simulink model "Trabajo_final_PID"  (R2020a)
settings: Solver=VariableStepAuto  StartTime=0.0  StopTime=2.1  MaxStep=Ts3  RelTol=1e-3
values from neighbouring files (symbols this model uses):
  b_1 = 0    [param.m]
  b_2 = 0    [param.m]
  b_3 = 0    [param.m]
  b_4 = 0    [param.m]
  ba_1 = J_1 * omega_b * n    (= 0.00155)    [param.m]
  ba_2 = J_2 * omega_b * n    (= 0.00155)    [param.m]
  ba_3 = J_3 * omega_b * n    (= 0.000516666666667)    [param.m]
  ba_4 = J_4 * omega_b * n    (= 0.00031)    [param.m]
  J_1 = Jl    (= 3.1e-06)    [param.m]
  J_2 = Jl    (= 3.1e-06)    [param.m]
  J_3 = Jl/3    (= 1.03333333333e-06)    [param.m]
  J_4 = Jl/5    (= 6.2e-07)    [param.m]
  Ke_omega_1 = 3*(polo^2)    (= 1920000)    [param.m]
  Ke_omega_2 = 3*(polo^2)    (= 1920000)    [param.m]
  Ke_omega_3 = 3*(polo^2)    (= 1920000)    [param.m]
  Ke_omega_4 = 3*(polo^2)    (= 1920000)    [param.m]
  Ke_tita_1 = 3*polo    (= 2400)    [param.m]
  Ke_tita_2 = 3*polo    (= 2400)    [param.m]
  Ke_tita_3 = 3*polo    (= 2400)    [param.m]
  Ke_tita_4 = 3*polo    (= 2400)    [param.m]
  Ke_zeta_1 = polo^3    (= 512000000)    [param.m]
  Ke_zeta_2 = polo^3    (= 512000000)    [param.m]
  Ke_zeta_3 = polo^3    (= 512000000)    [param.m]
  Ke_zeta_4 = polo^3    (= 512000000)    [param.m]
  Ksa_1 = J_1 *n *omega_b^2    (= 0.31)    [param.m]
  Ksa_2 = J_2 *n *omega_b^2    (= 0.31)    [param.m]
  Ksa_3 = J_3 *n *omega_b^2    (= 0.103333333333)    [param.m]
  Ksa_4 = J_4 *n *omega_b^2    (= 0.062)    [param.m]
  Ksia_1 = J_1*omega_b^3    (= 24.8)    [param.m]
  Ksia_2 = J_2*omega_b^3    (= 24.8)    [param.m]
  Ksia_3 = J_3*omega_b^3    (= 8.26666666667)    [param.m]
  Ksia_4 = J_4*omega_b^3    (= 4.96)    [param.m]
  r1 = 71.2    [param.m]
  r2 = 99.5    [param.m]
  r3 = 171    [param.m]
  r4 = 298    [param.m]
  Ts1 = (omega_b*25/(2*pi))^(-1)    (= 0.00125663706144)    [param.m]
  Ts2 = (polo*25/(2*pi))^(-1)    (= 0.000314159265359)    [param.m]
undefined symbols (not defined in the file or in its folder): DiscIntNeverNeededParam
libraries: dspstat3 x8, robotmaniplib x7, simulink x2
settings Model: Creator=Rodrigo  LastModifiedBy=Rodrigo

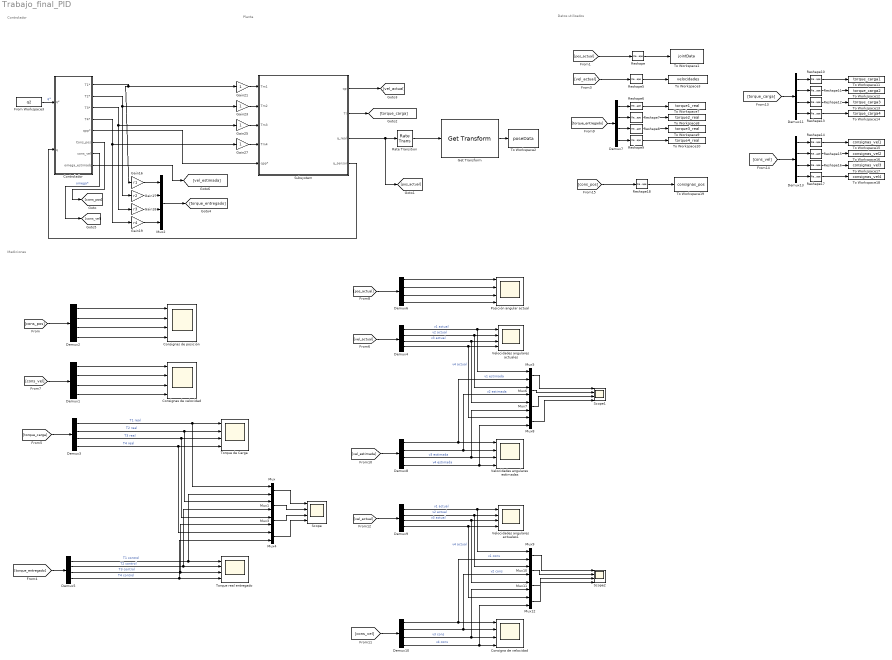
== system Trabajo_final_PID ==
  note: Planta
  note: Controlador
  note: Datos utilizados
  note: Mediciones
  "Consigna de velocidad " : Scope  NumInputPorts=4
  Consignas de posición : Scope  NumInputPorts=4
  Consignas de velocidad : Scope  NumInputPorts=4
  Controlador : Subsystem
  Demux{1..11,13} (12 alike) : Demux
  From Workspace3 : FromWorkspace  VariableName=q2  SampleTime=Ts2
  Gain16 : Gain  Gain=r1
  Gain17 : Gain  Gain=r2
  Gain18 : Gain  Gain=r3
  Gain19 : Gain  Gain=r4
  Gain{21,23,25,27} (4 alike) : Gain
  Get Transform : robotmaniplib/Get Transform  RigidBodyTree=robot  SourceBody=tool  TargetBody=base_link  SimulateUsing=Interpreted execution
  Mux{,1,3..12} (12 alike) : Mux  Inputs=2
  Mux2 : Mux
  Posición angular actual : Scope  NumInputPorts=4
  Rate Transition : RateTransition
  Reshape{,5..18} (15 alike) : Reshape
  Scope : Scope  NumInputPorts=4
  Scope1 : Scope  NumInputPorts=4
  Scope2 : Scope  NumInputPorts=4
  Subsystem : Subsystem
  To Workspace1 : ToWorkspace  VariableName=jointData  SampleTime=-1
      settings: Save2DSignal=2-D array (concatenate along first dimension)
  To Workspace10 : ToWorkspace  VariableName=torque4_real  SaveFormat=Timeseries  SampleTime=-1
  To Workspace11 : ToWorkspace  VariableName=torque_carga1  SaveFormat=Timeseries  SampleTime=-1
  To Workspace12 : ToWorkspace  VariableName=torque_carga2  SaveFormat=Timeseries  SampleTime=-1
  To Workspace13 : ToWorkspace  VariableName=torque_carga3  SaveFormat=Timeseries  SampleTime=-1
  To Workspace14 : ToWorkspace  VariableName=torque_carga4  SaveFormat=Timeseries  SampleTime=-1
  To Workspace15 : ToWorkspace  VariableName=consignas_vel1  SaveFormat=Timeseries  SampleTime=-1
  To Workspace16 : ToWorkspace  VariableName=consignas_vel2  SaveFormat=Timeseries  SampleTime=-1
  To Workspace17 : ToWorkspace  VariableName=consignas_vel3  SaveFormat=Timeseries  SampleTime=-1
  To Workspace18 : ToWorkspace  VariableName=consignas_vel4  SaveFormat=Timeseries  SampleTime=-1
  To Workspace19 : ToWorkspace  VariableName=consignas_pos  SampleTime=-1
      settings: Save2DSignal=2-D array (concatenate along first dimension)
  To Workspace2 : ToWorkspace  VariableName=poseData  SampleTime=-1
  To Workspace3 : ToWorkspace  VariableName=velocidades  SampleTime=-1
      settings: Save2DSignal=2-D array (concatenate along first dimension)
  To Workspace7 : ToWorkspace  VariableName=torque1_real  SaveFormat=Timeseries  SampleTime=-1
  To Workspace8 : ToWorkspace  VariableName=torque2_real  SaveFormat=Timeseries  SampleTime=-1
  To Workspace9 : ToWorkspace  VariableName=torque3_real  SaveFormat=Timeseries  SampleTime=-1
  Torque de Carga : Scope  NumInputPorts=4
  Torque real entregado : Scope  NumInputPorts=4
  Velocidades angulares actuales : Scope  NumInputPorts=4
  Velocidades angulares actuales1 : Scope  NumInputPorts=4
  Velocidades angulares estimadas : Scope  NumInputPorts=4
  wires:
  Rate Transition/1 -> Get Transform/1
  Get Transform/1 -> To Workspace2/1
  Demux2/1 -> Consignas de posición/1
  Demux2/2 -> Consignas de posición/2
  Demux2/3 -> Consignas de posición/3
  Demux2/4 -> Consignas de posición/4
  [cons_pos] -> Demux2/1
  Reshape/1 -> To Workspace1/1
  [pos_actual] -> Reshape/1
  Reshape5/1 -> To Workspace3/1
  [vel_actual] -> Reshape5/1
  Mux2/1 -> [torque_entregado]
  [torque_carga] -> Demux3/1
  Demux3/2 -> Torque de Carga/2, Mux1/1  "T2 real"
  Demux3/1 -> Torque de Carga/1, Mux/1  "T1 real"
  Demux3/3 -> Torque de Carga/3, Mux3/1  "T3 real"
  Demux3/4 -> Mux4/1, Torque de Carga/4  "T4 real"
  [vel_actual] -> Demux4/1
  Demux4/1 -> Mux5/1, Velocidades angulares actuales/1  "v1 actual"
  Demux4/2 -> Mux6/1, Velocidades angulares actuales/2  "v2 actual"
  Demux4/3 -> Mux7/1, Velocidades angulares actuales/3  "v3 actual"
  Demux4/4 -> Mux8/1, Velocidades angulares actuales/4  "v4 actual"
  [torque_entregado] -> Demux5/1
  Demux5/1 -> Torque real entregado/1, Mux/2  "T1 control"
  Demux5/2 -> Torque real entregado/2, Mux1/2  "T2 control"
  Demux5/3 -> Torque real entregado/3, Mux3/2  "T3 control"
  Demux5/4 -> Mux4/2, Torque real entregado/4  "T4 control"
  [cons_vel] -> Demux1/1
  Demux1/1 -> Consignas de velocidad/1
  Demux1/3 -> Consignas de velocidad/3
  Demux1/2 -> Consignas de velocidad/2
  Demux1/4 -> Consignas de velocidad/4
  Demux6/2 -> Posición angular actual/2
  [pos_actual] -> Demux6/1
  Demux6/4 -> Posición angular actual/4
  Demux6/1 -> Posición angular actual/1
  Demux6/3 -> Posición angular actual/3
  Reshape8/1 -> To Workspace9/1
  Demux7/2 -> Reshape7/1
  Demux7/4 -> Reshape9/1
  Reshape7/1 -> To Workspace8/1
  Reshape6/1 -> To Workspace7/1
  Reshape9/1 -> To Workspace10/1
  Demux7/1 -> Reshape6/1
  Demux7/3 -> Reshape8/1
  [torque_entregado] -> Demux7/1
  Gain19/1 -> Mux2/4
  Gain18/1 -> Mux2/3
  Gain17/1 -> Mux2/2
  Gain16/1 -> Mux2/1
  Gain25/1 -> Subsystem/3(Tm3)
  Gain27/1 -> Subsystem/4(Tm4)
  Gain23/1 -> Subsystem/2(Tm2)
  Gain21/1 -> Subsystem/1(Tm1)
  Subsystem/1(qp) -> [vel_actual]
  Subsystem/2(Tl) -> [torque_carga]
  Subsystem/3(q_real) -> [pos_actual], Rate Transition/1
  Controlador/4(T4*) -> Gain27/1, Gain19/1
  Controlador/3(T3*) -> Gain25/1, Gain18/1
  From Workspace3/1 -> Controlador/1(q*)  "q*"
  Controlador/2(T2*) -> Gain17/1, Gain23/1
  Controlador/5(qpp*) -> Subsystem/5(qpp*)
  Controlador/6(Cons_pos) -> [cons_pos]
  Controlador/7(cons_vel) -> [cons_vel]  "omega*"
  Controlador/1(T1*) -> Gain21/1, Gain16/1
  Mux/1 -> Scope/1
  Mux1/1 -> Scope/2
  Mux3/1 -> Scope/3
  Mux4/1 -> Scope/4
  Controlador/8(omega_estimado) -> [vel_estimada]
  Demux8/4 -> Mux8/2, Velocidades angulares estimadas/4  "v4 estimada"
  [vel_estimada] -> Demux8/1
  Demux8/2 -> Velocidades angulares estimadas/2, Mux6/2  "v2 estimada"
  Demux8/3 -> Mux7/2, Velocidades angulares estimadas/3  "v3 estimada"
  Demux8/1 -> Velocidades angulares estimadas/1, Mux5/2  "v1 estimada"
  Mux8/1 -> Scope1/4
  Mux7/1 -> Scope1/3
  Mux5/1 -> Scope1/1
  Mux6/1 -> Scope1/2
  [cons_vel] -> Demux10/1
  Demux10/1 -> "Consigna de velocidad "/1, Mux9/2  "v1 cons"
  Demux10/3 -> Mux11/2, "Consigna de velocidad "/3  "v3 cons"
  Demux10/4 -> Mux12/2, "Consigna de velocidad "/4  "v4 cons"
  Mux12/1 -> Scope2/4
  Demux10/2 -> "Consigna de velocidad "/2, Mux10/2  "v2 cons"
  Mux9/1 -> Scope2/1
  [vel_actual] -> Demux9/1
  Mux11/1 -> Scope2/3
  Demux9/3 -> Mux11/1, Velocidades angulares actuales1/3  "v3 actual"
  Demux9/2 -> Mux10/1, Velocidades angulares actuales1/2  "v2 actual"
  Demux9/1 -> Mux9/1, Velocidades angulares actuales1/1  "v1 actual"
  Mux10/1 -> Scope2/2
  Demux9/4 -> Mux12/1, Velocidades angulares actuales1/4  "v4 actual"
  Subsystem/4(q_sensor) -> Controlador/2(q)
  Reshape11/1 -> To Workspace12/1
  Reshape12/1 -> To Workspace13/1
  Demux11/2 -> Reshape11/1
  [torque_carga] -> Demux11/1
  Reshape10/1 -> To Workspace11/1
  Reshape13/1 -> To Workspace14/1
  Demux11/4 -> Reshape13/1
  Demux11/1 -> Reshape10/1
  Demux11/3 -> Reshape12/1
  Demux13/2 -> Reshape15/1
  Reshape14/1 -> To Workspace15/1
  Demux13/3 -> Reshape16/1
  [cons_vel] -> Demux13/1
  Reshape17/1 -> To Workspace18/1
  Reshape15/1 -> To Workspace16/1
  Demux13/1 -> Reshape14/1
  Demux13/4 -> Reshape17/1
  Reshape16/1 -> To Workspace17/1
  [cons_pos] -> Reshape18/1
  Reshape18/1 -> To Workspace19/1

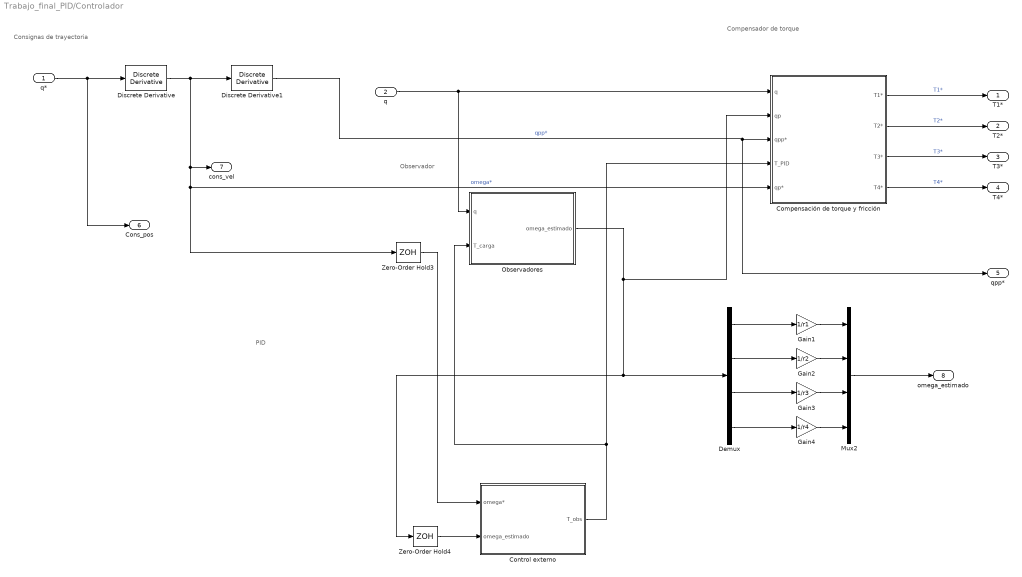
== system Trabajo_final_PID/Controlador ==
  note: Compensador de torque
  note: Observador
  note: PID
  note: Consignas de trayectoria
  q* : Inport
  q : Inport  Port=2
  Compensación de torque y fricción : Subsystem
  Control externo : Subsystem
  Demux : Demux
  Discrete Derivative : simulink/Discrete/Discrete Derivative  gainval=1.0  ICPrevScaledInput=0.0  OutMin=[]  OutMax=[]  OutDataType=fixdt(1, 16)  OutScaling=2^-10  DoSatur=off
  Discrete Derivative1 : simulink/Discrete/Discrete Derivative  gainval=1.0  ICPrevScaledInput=0.0  OutMin=[]  OutMax=[]  OutDataType=fixdt(1, 16)  OutScaling=2^-10  DoSatur=off
  Gain1 : Gain  Gain=1/r1
  Gain2 : Gain  Gain=1/r2
  Gain3 : Gain  Gain=1/r3
  Gain4 : Gain  Gain=1/r4
  Mux2 : Mux
  Observadores : Subsystem
  Zero-Order Hold3 : ZeroOrderHold  SampleTime=Ts1
  Zero-Order Hold4 : ZeroOrderHold  SampleTime=Ts1
  T1* : Outport
  T2* : Outport  Port=2
  T3* : Outport  Port=3
  T4* : Outport  Port=4
  qpp* : Outport  Port=5
  Cons_pos : Outport  Port=6
  cons_vel : Outport  Port=7
  omega_estimado : Outport  Port=8
  wires:
  Discrete Derivative/1 -> cons_vel/1, Zero-Order Hold3/1, Compensación de torque y fricción/5(qp*), Discrete Derivative1/1  "omega*"
  q/1 -> Compensación de torque y fricción/1(q), Observadores/1(q)
  Control externo/1(T_obs) -> Compensación de torque y fricción/4(T_PID), Observadores/2(T_carga)
  Discrete Derivative1/1 -> qpp*/1, Compensación de torque y fricción/3(qpp*)  "qpp*"
  Zero-Order Hold3/1 -> Control externo/1(omega*)
  Zero-Order Hold4/1 -> Control externo/2(omega_estimado)
  Compensación de torque y fricción/2(T2*) -> T2*/1  "T2*"
  Observadores/1(omega_estimado) -> Demux/1, Zero-Order Hold4/1, Compensación de torque y fricción/2(qp)
  Compensación de torque y fricción/4(T4*) -> T4*/1  "T4*"
  Compensación de torque y fricción/3(T3*) -> T3*/1  "T3*"
  Compensación de torque y fricción/1(T1*) -> T1*/1  "T1*"
  q*/1 -> Cons_pos/1, Discrete Derivative/1
  Gain2/1 -> Mux2/2
  Mux2/1 -> omega_estimado/1
  Gain1/1 -> Mux2/1
  Gain4/1 -> Mux2/4
  Gain3/1 -> Mux2/3
  Demux/1 -> Gain1/1
  Demux/2 -> Gain2/1
  Demux/3 -> Gain3/1
  Demux/4 -> Gain4/1

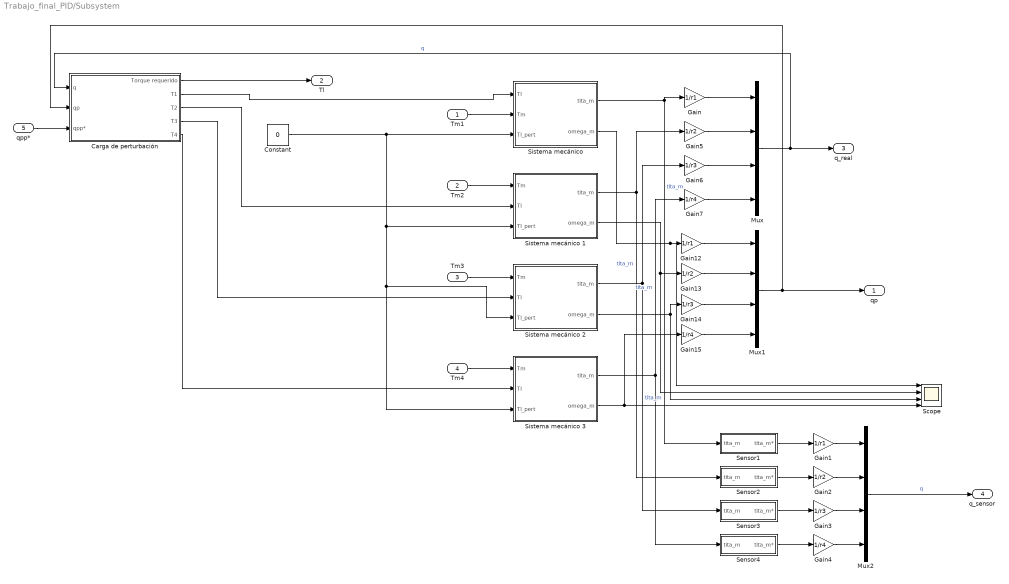
== system Trabajo_final_PID/Subsystem ==
  Tm1 : Inport
  Tm2 : Inport  Port=2
  Tm3 : Inport  Port=3
  Tm4 : Inport  Port=4
  qpp* : Inport  Port=5
  Carga de perturbación : Subsystem
  Constant : Constant  Value=0
  Gain : Gain  Gain=1/r1
  Gain1 : Gain  Gain=1/r1
  Gain12 : Gain  Gain=1/r1
  Gain13 : Gain  Gain=1/r2
  Gain14 : Gain  Gain=1/r3
  Gain15 : Gain  Gain=1/r4
  Gain2 : Gain  Gain=1/r2
  Gain3 : Gain  Gain=1/r3
  Gain4 : Gain  Gain=1/r4
  Gain5 : Gain  Gain=1/r2
  Gain6 : Gain  Gain=1/r3
  Gain7 : Gain  Gain=1/r4
  Mux : Mux
  Mux1 : Mux
  Mux2 : Mux
  Scope : Scope  NumInputPorts=4
  Sensor1 : Subsystem
  Sensor2 : Subsystem
  Sensor3 : Subsystem
  Sensor4 : Subsystem
  "Sistema mecánico " : Subsystem
  Sistema mecánico 1 : Subsystem
  Sistema mecánico 2 : Subsystem
  Sistema mecánico 3 : Subsystem
  qp : Outport
  Tl : Outport  Port=2
  q_real : Outport  Port=3
  q_sensor : Outport  Port=4
  wires:
  Gain13/1 -> Mux1/2
  Gain5/1 -> Mux/2
  Sistema mecánico 3/2(omega_m) -> Gain15/1, Scope/4
  Gain15/1 -> Mux1/4
  Sistema mecánico 3/1(tita_m) -> Sensor4/1(tita_m), Gain7/1  "tita_m"
  Mux/1 -> q_real/1, Carga de perturbación/1(q)  "q"
  Tm1/1 -> "Sistema mecánico "/2(Tm)
  Sistema mecánico 1/2(omega_m) -> Scope/2, Gain13/1
  Tm4/1 -> Sistema mecánico 3/1(Tm)
  "Sistema mecánico "/2(omega_m) -> Scope/1, Gain12/1
  Sistema mecánico 1/1(tita_m) -> Sensor2/1(tita_m), Gain5/1  "tita_m"
  Sistema mecánico 2/2(omega_m) -> Gain14/1, Scope/3
  Gain12/1 -> Mux1/1
  Gain14/1 -> Mux1/3
  Gain7/1 -> Mux/4
  Gain/1 -> Mux/1
  Gain6/1 -> Mux/3
  Sistema mecánico 2/1(tita_m) -> Sensor3/1(tita_m), Gain6/1  "tita_m"
  "Sistema mecánico "/1(tita_m) -> Gain/1, Sensor1/1(tita_m)  "tita_m"
  Tm3/1 -> Sistema mecánico 2/1(Tm)
  Tm2/1 -> Sistema mecánico 1/1(Tm)
  Carga de perturbación/2(T1) -> "Sistema mecánico "/1(Tl)
  Carga de perturbación/3(T2) -> Sistema mecánico 1/2(Tl)
  Carga de perturbación/4(T3) -> Sistema mecánico 2/2(Tl)
  Carga de perturbación/5(T4) -> Sistema mecánico 3/2(Tl)
  Carga de perturbación/1(Torque requerido) -> Tl/1
  Mux1/1 -> Carga de perturbación/2(qp), qp/1
  qpp*/1 -> Carga de perturbación/3(qpp*)
  Gain1/1 -> Mux2/1
  Sensor1/1(tita_m*) -> Gain1/1
  Gain2/1 -> Mux2/2
  Gain3/1 -> Mux2/3
  Gain4/1 -> Mux2/4
  Sensor4/1(tita_m*) -> Gain4/1
  Sensor3/1(tita_m*) -> Gain3/1
  Sensor2/1(tita_m*) -> Gain2/1
  Mux2/1 -> q_sensor/1  "q"
  Constant/1 -> Sistema mecánico 3/3(Tl_pert), Sistema mecánico 2/3(Tl_pert), Sistema mecánico 1/3(Tl_pert), "Sistema mecánico "/3(Tl_pert)

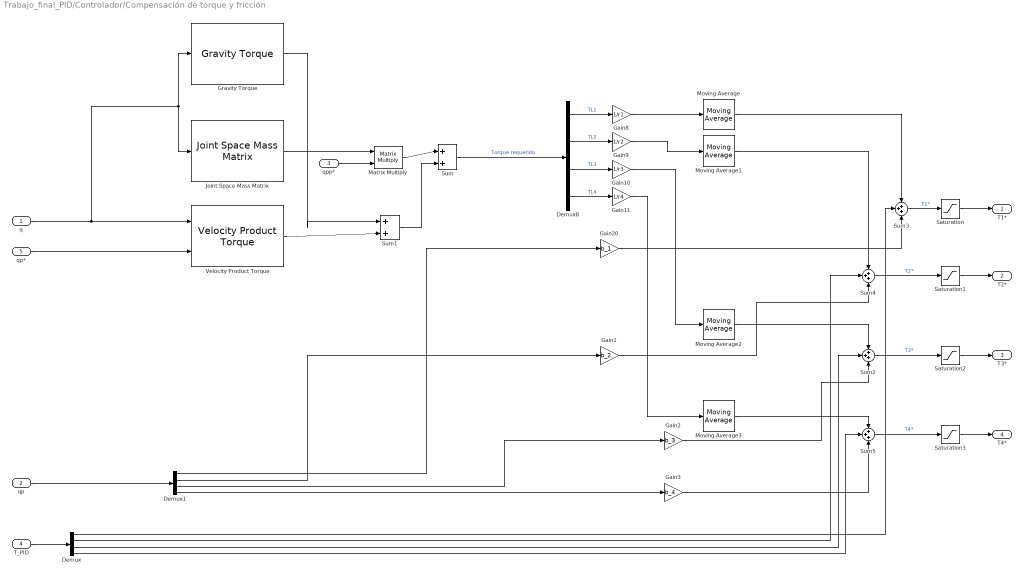
== system Trabajo_final_PID/Controlador/Compensación de torque y fricción ==
  q : Inport
  qp : Inport  Port=2
  qpp* : Inport  Port=3
  T_PID : Inport  Port=4
  qp* : Inport  Port=5
  Demux : Demux
  Demux1 : Demux
  Demux8 : Demux
  Gain1 : Gain  Gain=b_2
  Gain10 : Gain  Gain=1/r3
  Gain11 : Gain  Gain=1/r4
  Gain2 : Gain  Gain=b_3
  Gain20 : Gain  Gain=b_1
  Gain3 : Gain  Gain=b_4
  Gain8 : Gain  Gain=1/r1
  Gain9 : Gain  Gain=1/r2
  Gravity Torque : robotmaniplib/Gravity Torque  RigidBodyTree=robot  SimulateUsing=Interpreted execution
  Joint Space Mass Matrix : robotmaniplib/Joint Space Mass Matrix  RigidBodyTree=robot  SimulateUsing=Interpreted execution
  Matrix Multiply : Product  Multiplication=Matrix(*)
  Moving Average{,1..3} (4 alike) : dspstat3/Moving Average  Method=Sliding window  ForgettingFactorPort=off  SpecifyWindowLength=on  WindowLength=5  ForgettingFactor=0.9  SimulateUsing=Code generation
  Saturation : Saturate  UpperLimit=10/r1  LowerLimit=-10/r1
  Saturation1 : Saturate  UpperLimit=8.2/r2  LowerLimit=-8.2/r2
  Saturation2 : Saturate  UpperLimit=3/r3  LowerLimit=-3/r3
  Saturation3 : Saturate  UpperLimit=0.8/r4  LowerLimit=-0.8/r4
  Sum : Sum  Inputs=|++
  Sum1 : Sum  Inputs=|++
  Sum{2..5} (4 alike) : Sum  Inputs=+++
  Velocity Product Torque : robotmaniplib/Velocity Product Torque  RigidBodyTree=robot  SimulateUsing=Interpreted execution
      settings: SourceProductBaseCode=RO
  T1* : Outport
  T2* : Outport  Port=2
  T3* : Outport  Port=3
  T4* : Outport  Port=4
  wires:
  q/1 -> Velocity Product Torque/1, Gravity Torque/1, Joint Space Mass Matrix/1
  Demux8/1 -> Gain8/1  "TL1"
  Matrix Multiply/1 -> Sum/1
  Sum/1 -> Demux8/1  "Torque requerido"
  Gravity Torque/1 -> Sum1/1
  Velocity Product Torque/1 -> Sum1/2
  Joint Space Mass Matrix/1 -> Matrix Multiply/1
  Sum1/1 -> Sum/2
  Demux8/4 -> Gain11/1  "TL4"
  Demux8/3 -> Gain10/1  "TL3"
  Demux8/2 -> Gain9/1  "TL2"
  qpp*/1 -> Matrix Multiply/2
  qp/1 -> Demux1/1
  Sum2/1 -> Saturation2/1  "T3*"
  Saturation2/1 -> T3*/1
  Gain10/1 -> Moving Average2/1
  Gain9/1 -> Moving Average1/1
  Saturation1/1 -> T2*/1
  Sum3/1 -> Saturation/1  "T1*"
  Sum4/1 -> Saturation1/1  "T2*"
  Saturation/1 -> T1*/1
  Demux/1 -> Sum3/2
  Sum5/1 -> Saturation3/1  "T4*"
  Gain8/1 -> Moving Average/1
  Gain11/1 -> Moving Average3/1
  Saturation3/1 -> T4*/1
  Gain20/1 -> Sum3/3
  Gain1/1 -> Sum4/3
  Gain2/1 -> Sum2/3
  Gain3/1 -> Sum5/3
  Demux1/1 -> Gain20/1
  Demux1/2 -> Gain1/1
  Demux1/3 -> Gain2/1
  Demux1/4 -> Gain3/1
  Demux/2 -> Sum4/2
  Demux/3 -> Sum2/2
  Demux/4 -> Sum5/2
  T_PID/1 -> Demux/1
  Moving Average/1 -> Sum3/1
  Moving Average1/1 -> Sum4/1
  Moving Average2/1 -> Sum2/1
  Moving Average3/1 -> Sum5/1
  qp*/1 -> Velocity Product Torque/2

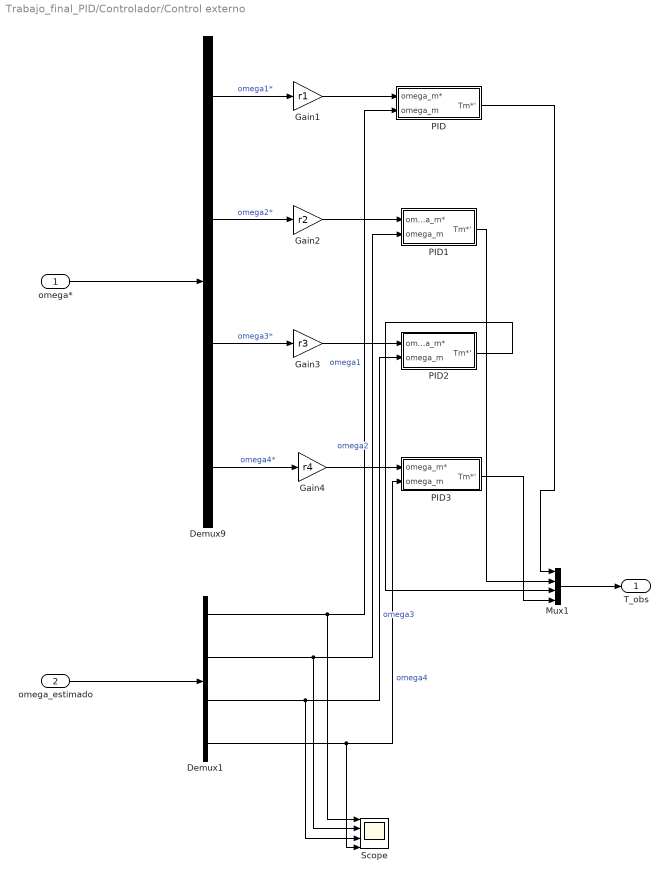
== system Trabajo_final_PID/Controlador/Control externo ==
  omega* : Inport
  omega_estimado : Inport  Port=2
  Demux1 : Demux
  Demux9 : Demux
  Gain1 : Gain  Gain=r1
  Gain2 : Gain  Gain=r2
  Gain3 : Gain  Gain=r3
  Gain4 : Gain  Gain=r4
  Mux1 : Mux
  PID : Subsystem
  PID1 : Subsystem
  PID2 : Subsystem
  PID3 : Subsystem
  Scope : Scope  NumInputPorts=4
  T_obs : Outport
  wires:
  Demux9/3 -> Gain3/1  "omega3*"
  Gain2/1 -> PID1/1(omega_m*)
  Gain3/1 -> PID2/1(omega_m*)
  Demux9/1 -> Gain1/1  "omega1*"
  Demux9/2 -> Gain2/1  "omega2*"
  Gain4/1 -> PID3/1(omega_m*)
  Demux9/4 -> Gain4/1  "omega4*"
  Gain1/1 -> PID/1(omega_m*)
  Demux1/2 -> Scope/2, PID1/2(omega_m)  "omega2"
  Demux1/1 -> Scope/1, PID/2(omega_m)  "omega1"
  Demux1/3 -> Scope/3, PID2/2(omega_m)  "omega3"
  Demux1/4 -> Scope/4, PID3/2(omega_m)  "omega4"
  PID/1(Tm*') -> Mux1/1
  PID1/1(Tm*') -> Mux1/2
  PID2/1(Tm*') -> Mux1/3
  PID3/1(Tm*') -> Mux1/4
  Mux1/1 -> T_obs/1
  omega*/1 -> Demux9/1
  omega_estimado/1 -> Demux1/1

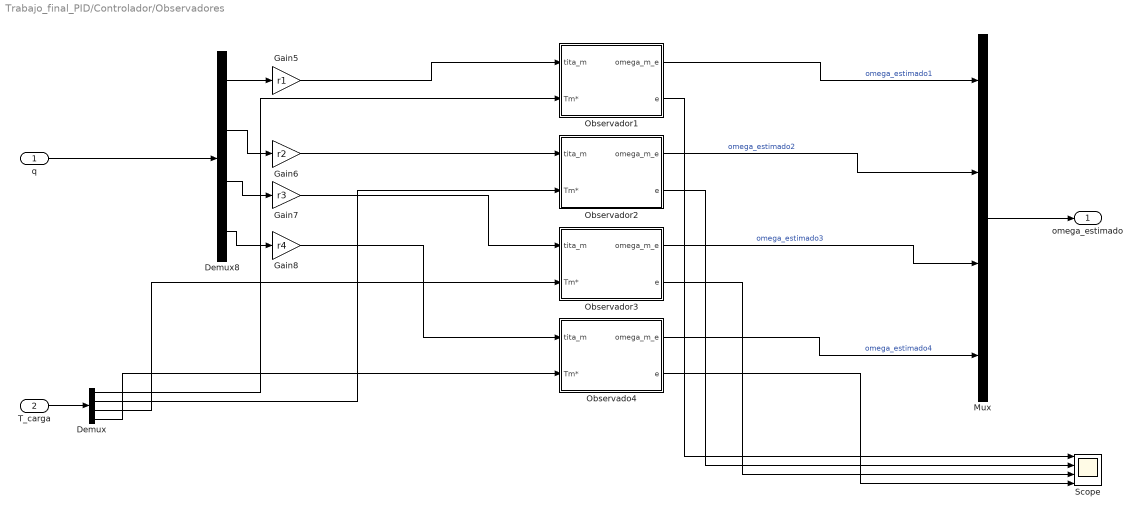
== system Trabajo_final_PID/Controlador/Observadores ==
  q : Inport
  T_carga : Inport  Port=2
  Demux : Demux
  Demux8 : Demux
  Gain5 : Gain  Gain=r1
  Gain6 : Gain  Gain=r2
  Gain7 : Gain  Gain=r3
  Gain8 : Gain  Gain=r4
  Mux : Mux
  Observado4 : Subsystem
  Observador1 : Subsystem
  Observador2 : Subsystem
  Observador3 : Subsystem
  Scope : Scope  NumInputPorts=4
  omega_estimado : Outport
  wires:
  Gain6/1 -> Observador2/1(tita_m)
  Demux8/3 -> Gain7/1
  Gain5/1 -> Observador1/1(tita_m)
  Demux8/1 -> Gain5/1
  Observador2/1(omega_m_e) -> Mux/2  "omega_estimado2"
  Demux8/2 -> Gain6/1
  Demux8/4 -> Gain8/1
  Gain7/1 -> Observador3/1(tita_m)
  Gain8/1 -> Observado4/1(tita_m)
  Observador1/1(omega_m_e) -> Mux/1  "omega_estimado1"
  Observado4/1(omega_m_e) -> Mux/4  "omega_estimado4"
  Observador3/1(omega_m_e) -> Mux/3  "omega_estimado3"
  q/1 -> Demux8/1
  Mux/1 -> omega_estimado/1
  T_carga/1 -> Demux/1
  Demux/1 -> Observador1/2(Tm*)
  Demux/2 -> Observador2/2(Tm*)
  Demux/3 -> Observador3/2(Tm*)
  Demux/4 -> Observado4/2(Tm*)
  Observador1/2(e) -> Scope/1
  Observador2/2(e) -> Scope/2
  Observador3/2(e) -> Scope/3
  Observado4/2(e) -> Scope/4

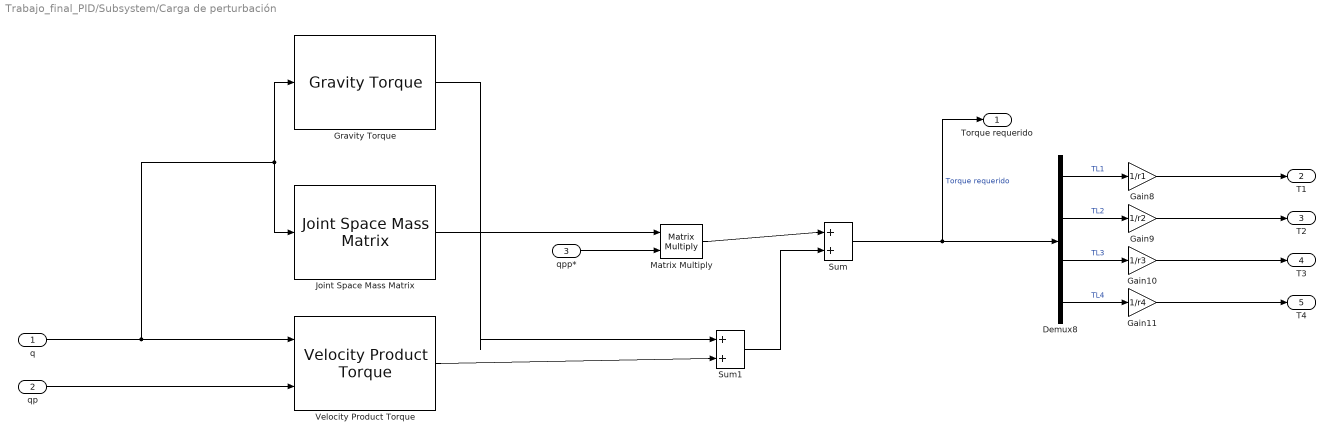
== system Trabajo_final_PID/Subsystem/Carga de perturbación ==
  q : Inport
  qp : Inport  Port=2
  qpp* : Inport  Port=3
  Demux8 : Demux
  Gain10 : Gain  Gain=1/r3
  Gain11 : Gain  Gain=1/r4
  Gain8 : Gain  Gain=1/r1
  Gain9 : Gain  Gain=1/r2
  Gravity Torque : robotmaniplib/Gravity Torque  RigidBodyTree=robot  SimulateUsing=Interpreted execution
  Joint Space Mass Matrix : robotmaniplib/Joint Space Mass Matrix  RigidBodyTree=robot  SimulateUsing=Interpreted execution
  Matrix Multiply : Product  Multiplication=Matrix(*)
  Sum : Sum  Inputs=|++
  Sum1 : Sum  Inputs=|++
  Velocity Product Torque : robotmaniplib/Velocity Product Torque  RigidBodyTree=robot  SimulateUsing=Interpreted execution
      settings: SourceProductBaseCode=RO
  Torque requerido : Outport
  T1 : Outport  Port=2
  T2 : Outport  Port=3
  T3 : Outport  Port=4
  T4 : Outport  Port=5
  wires:
  q/1 -> Velocity Product Torque/1, Gravity Torque/1, Joint Space Mass Matrix/1
  Demux8/1 -> Gain8/1  "TL1"
  Matrix Multiply/1 -> Sum/1
  Sum/1 -> Demux8/1, Torque requerido/1  "Torque requerido"
  Gravity Torque/1 -> Sum1/1
  Velocity Product Torque/1 -> Sum1/2
  Joint Space Mass Matrix/1 -> Matrix Multiply/1
  Sum1/1 -> Sum/2
  Demux8/4 -> Gain11/1  "TL4"
  Demux8/3 -> Gain10/1  "TL3"
  Gain11/1 -> T4/1
  Demux8/2 -> Gain9/1  "TL2"
  qpp*/1 -> Matrix Multiply/2
  qp/1 -> Velocity Product Torque/2
  Gain9/1 -> T2/1
  Gain8/1 -> T1/1
  Gain10/1 -> T3/1

== system Trabajo_final_PID/Subsystem/Sensor1 ==
  tita_m : Inport
  Moving Average : dspstat3/Moving Average  Method=Sliding window  ForgettingFactorPort=off  SpecifyWindowLength=on  WindowLength=8  ForgettingFactor=0.9  SimulateUsing=Code generation
  Quantizer : Quantizer  QuantizationInterval=int_encoder
  Random Number : RandomNumber  Variance=(1/360)^2  SampleTime=Ts2  VectorParams1D=off
  Sum : Sum  Inputs=|++
  Zero-Order Hold1 : ZeroOrderHold  SampleTime=Ts2
  tita_m* : Outport
  wires:
  tita_m/1 -> Quantizer/1
  Random Number/1 -> Sum/2
  Zero-Order Hold1/1 -> Moving Average/1  "tita_m*"
  Moving Average/1 -> tita_m*/1
  Sum/1 -> Zero-Order Hold1/1
  Quantizer/1 -> Sum/1

== system Trabajo_final_PID/Subsystem/Sensor2 ==
  tita_m : Inport
  Moving Average : dspstat3/Moving Average  Method=Sliding window  ForgettingFactorPort=off  SpecifyWindowLength=on  WindowLength=8  ForgettingFactor=0.9  SimulateUsing=Code generation
  Quantizer : Quantizer  QuantizationInterval=int_encoder
  Random Number : RandomNumber  Variance=(1/360)^2  SampleTime=Ts2  VectorParams1D=off
  Sum : Sum  Inputs=|++
  Zero-Order Hold1 : ZeroOrderHold  SampleTime=Ts2
  tita_m* : Outport
  wires:
  tita_m/1 -> Quantizer/1
  Random Number/1 -> Sum/2
  Sum/1 -> Zero-Order Hold1/1
  Zero-Order Hold1/1 -> Moving Average/1  "tita_m*"
  Moving Average/1 -> tita_m*/1
  Quantizer/1 -> Sum/1

== system Trabajo_final_PID/Subsystem/Sensor3 ==
  tita_m : Inport
  Moving Average : dspstat3/Moving Average  Method=Sliding window  ForgettingFactorPort=off  SpecifyWindowLength=on  WindowLength=8  ForgettingFactor=0.9  SimulateUsing=Code generation
  Quantizer : Quantizer  QuantizationInterval=int_encoder
  Random Number : RandomNumber  Variance=(1/360)^2  SampleTime=Ts2  VectorParams1D=off
  Sum : Sum  Inputs=|++
  Zero-Order Hold1 : ZeroOrderHold  SampleTime=Ts2
  tita_m* : Outport
  wires:
  tita_m/1 -> Quantizer/1
  Random Number/1 -> Sum/2
  Sum/1 -> Zero-Order Hold1/1
  Zero-Order Hold1/1 -> Moving Average/1  "tita_m*"
  Moving Average/1 -> tita_m*/1
  Quantizer/1 -> Sum/1

== system Trabajo_final_PID/Subsystem/Sensor4 ==
  tita_m : Inport
  Moving Average : dspstat3/Moving Average  Method=Sliding window  ForgettingFactorPort=off  SpecifyWindowLength=on  WindowLength=8  ForgettingFactor=0.9  SimulateUsing=Code generation
  Quantizer : Quantizer  QuantizationInterval=int_encoder
  Random Number : RandomNumber  Variance=(1/360)^2  SampleTime=Ts2  VectorParams1D=off
  Sum : Sum  Inputs=|++
  Zero-Order Hold1 : ZeroOrderHold  SampleTime=Ts2
  tita_m* : Outport
  wires:
  tita_m/1 -> Quantizer/1
  Random Number/1 -> Sum/2
  Sum/1 -> Zero-Order Hold1/1
  Zero-Order Hold1/1 -> Moving Average/1  "tita_m*"
  Moving Average/1 -> tita_m*/1
  Quantizer/1 -> Sum/1

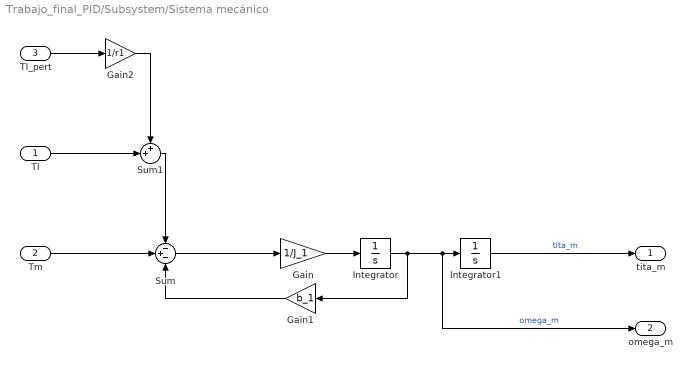
== system Trabajo_final_PID/Subsystem/Sistema mecánico  ==
  Tl : Inport
  Tm : Inport  Port=2
  Tl_pert : Inport  Port=3
  Gain : Gain  Gain=1/J_1
  Gain1 : Gain  Gain=b_1
  Gain2 : Gain  Gain=1/r1
  Integrator : Integrator
  Integrator1 : Integrator
  Sum : Sum  Inputs=-+-
  Sum1 : Sum  Inputs=++|
  tita_m : Outport  VectorParamsAs1DForOutWhenUnconnected=off
  omega_m : Outport  Port=2
  wires:
  Integrator/1 -> Gain1/1, omega_m/1, Integrator1/1  "omega_m"
  Sum/1 -> Gain/1
  Integrator1/1 -> tita_m/1  "tita_m"
  Tm/1 -> Sum/2
  Gain/1 -> Integrator/1
  Gain1/1 -> Sum/3
  Sum1/1 -> Sum/1
  Tl/1 -> Sum1/2
  Tl_pert/1 -> Gain2/1
  Gain2/1 -> Sum1/1

== system Trabajo_final_PID/Subsystem/Sistema mecánico 1 ==
  Tm : Inport
  Tl : Inport  Port=2
  Tl_pert : Inport  Port=3
  Gain : Gain  Gain=1/J_2
  Gain1 : Gain  Gain=b_2
  Gain2 : Gain  Gain=1/r2
  Integrator : Integrator
  Integrator1 : Integrator
  Sum : Sum  Inputs=-+-
  Sum1 : Sum  Inputs=++|
  tita_m : Outport  VectorParamsAs1DForOutWhenUnconnected=off
  omega_m : Outport  Port=2
  wires:
  Integrator/1 -> Gain1/1, omega_m/1, Integrator1/1  "omega_m"
  Sum/1 -> Gain/1
  Integrator1/1 -> tita_m/1  "tita_m"
  Tm/1 -> Sum/2
  Gain/1 -> Integrator/1
  Gain1/1 -> Sum/3
  Tl/1 -> Sum1/2
  Sum1/1 -> Sum/1
  Tl_pert/1 -> Gain2/1
  Gain2/1 -> Sum1/1

== system Trabajo_final_PID/Subsystem/Sistema mecánico 2 ==
  Tm : Inport
  Tl : Inport  Port=2
  Tl_pert : Inport  Port=3
  Gain : Gain  Gain=1/J_3
  Gain1 : Gain  Gain=b_3
  Gain2 : Gain  Gain=1/r3
  Integrator : Integrator
  Integrator1 : Integrator
  Sum : Sum  Inputs=-+-
  Sum1 : Sum  Inputs=++|
  tita_m : Outport  VectorParamsAs1DForOutWhenUnconnected=off
  omega_m : Outport  Port=2
  wires:
  Integrator/1 -> Gain1/1, omega_m/1, Integrator1/1  "omega_m"
  Sum/1 -> Gain/1
  Integrator1/1 -> tita_m/1  "tita_m"
  Tm/1 -> Sum/2
  Gain/1 -> Integrator/1
  Gain1/1 -> Sum/3
  Tl/1 -> Sum1/2
  Sum1/1 -> Sum/1
  Tl_pert/1 -> Gain2/1
  Gain2/1 -> Sum1/1

== system Trabajo_final_PID/Subsystem/Sistema mecánico 3 ==
  Tm : Inport
  Tl : Inport  Port=2
  Tl_pert : Inport  Port=3
  Gain : Gain  Gain=1/J_4
  Gain1 : Gain  Gain=b_2
  Gain2 : Gain  Gain=1/r4
  Integrator : Integrator
  Integrator1 : Integrator
  Sum : Sum  Inputs=-+-
  Sum1 : Sum  Inputs=++|
  tita_m : Outport  VectorParamsAs1DForOutWhenUnconnected=off
  omega_m : Outport  Port=2
  wires:
  Integrator/1 -> Gain1/1, omega_m/1, Integrator1/1  "omega_m"
  Sum/1 -> Gain/1
  Integrator1/1 -> tita_m/1  "tita_m"
  Tm/1 -> Sum/2
  Gain/1 -> Integrator/1
  Gain1/1 -> Sum/3
  Tl/1 -> Sum1/2
  Sum1/1 -> Sum/1
  Tl_pert/1 -> Gain2/1
  Gain2/1 -> Sum1/1

== system Trabajo_final_PID/Controlador/Control externo/PID ==
  omega_m* : Inport
  omega_m : Inport  Port=2
  Discrete-Time Integrator : DiscreteIntegrator  SampleTime=Ts1  ICPrevOutput=DiscIntNeverNeededParam  ICPrevScaledInput=DiscIntNeverNeededParam
  Discrete-Time Integrator1 : DiscreteIntegrator  SampleTime=Ts1  ICPrevOutput=DiscIntNeverNeededParam  ICPrevScaledInput=DiscIntNeverNeededParam
  Gain7 : Gain  Gain=ba_1
  Gain8 : Gain  Gain=Ksa_1
  Gain9 : Gain  Gain=Ksia_1
  Sum5 : Sum  Inputs=|+-
  Sum6 : Sum  Inputs=+++
  Tm*' : Outport  VectorParamsAs1DForOutWhenUnconnected=off
  wires:
  Gain8/1 -> Sum6/2
  Gain9/1 -> Sum6/1
  omega_m/1 -> Sum5/2
  Sum6/1 -> Tm*'/1  "Tm*'"
  Discrete-Time Integrator/1 -> Discrete-Time Integrator1/1, Gain8/1
  Discrete-Time Integrator1/1 -> Gain9/1
  Sum5/1 -> Gain7/1, Discrete-Time Integrator/1  "e_w"
  omega_m*/1 -> Sum5/1
  Gain7/1 -> Sum6/3

== system Trabajo_final_PID/Controlador/Control externo/PID1 ==
  omega_m* : Inport
  omega_m : Inport  Port=2
  Discrete-Time Integrator : DiscreteIntegrator  SampleTime=Ts1  ICPrevOutput=DiscIntNeverNeededParam  ICPrevScaledInput=DiscIntNeverNeededParam
  Discrete-Time Integrator1 : DiscreteIntegrator  SampleTime=Ts1  ICPrevOutput=DiscIntNeverNeededParam  ICPrevScaledInput=DiscIntNeverNeededParam
  Gain7 : Gain  Gain=ba_2
  Gain8 : Gain  Gain=Ksa_2
  Gain9 : Gain  Gain=Ksia_2
  Sum5 : Sum  Inputs=|+-
  Sum6 : Sum  Inputs=+++
  Tm*' : Outport  VectorParamsAs1DForOutWhenUnconnected=off
  wires:
  Gain8/1 -> Sum6/2
  Gain9/1 -> Sum6/1
  omega_m/1 -> Sum5/2
  Gain7/1 -> Sum6/3
  Sum6/1 -> Tm*'/1  "Tm*'"
  Discrete-Time Integrator/1 -> Discrete-Time Integrator1/1, Gain8/1
  Discrete-Time Integrator1/1 -> Gain9/1
  Sum5/1 -> Discrete-Time Integrator/1, Gain7/1  "e_w"
  omega_m*/1 -> Sum5/1

== system Trabajo_final_PID/Controlador/Control externo/PID2 ==
  omega_m* : Inport
  omega_m : Inport  Port=2
  Discrete-Time Integrator : DiscreteIntegrator  SampleTime=Ts1  ICPrevOutput=DiscIntNeverNeededParam  ICPrevScaledInput=DiscIntNeverNeededParam
  Discrete-Time Integrator1 : DiscreteIntegrator  SampleTime=Ts1  ICPrevOutput=DiscIntNeverNeededParam  ICPrevScaledInput=DiscIntNeverNeededParam
  Gain7 : Gain  Gain=ba_3
  Gain8 : Gain  Gain=Ksa_3
  Gain9 : Gain  Gain=Ksia_3
  Sum5 : Sum  Inputs=|+-
  Sum6 : Sum  Inputs=+++
  Tm*' : Outport  VectorParamsAs1DForOutWhenUnconnected=off
  wires:
  Gain8/1 -> Sum6/2
  Gain9/1 -> Sum6/1
  omega_m/1 -> Sum5/2
  Gain7/1 -> Sum6/3
  Sum6/1 -> Tm*'/1  "Tm*'"
  Discrete-Time Integrator/1 -> Discrete-Time Integrator1/1, Gain8/1
  Discrete-Time Integrator1/1 -> Gain9/1
  Sum5/1 -> Discrete-Time Integrator/1, Gain7/1  "e_w"
  omega_m*/1 -> Sum5/1

== system Trabajo_final_PID/Controlador/Control externo/PID3 ==
  omega_m* : Inport
  omega_m : Inport  Port=2
  Discrete-Time Integrator : DiscreteIntegrator  SampleTime=Ts1  ICPrevOutput=DiscIntNeverNeededParam  ICPrevScaledInput=DiscIntNeverNeededParam
  Discrete-Time Integrator1 : DiscreteIntegrator  SampleTime=Ts1  ICPrevOutput=DiscIntNeverNeededParam  ICPrevScaledInput=DiscIntNeverNeededParam
  Gain7 : Gain  Gain=ba_4
  Gain8 : Gain  Gain=Ksa_4
  Gain9 : Gain  Gain=Ksia_4
  Sum5 : Sum  Inputs=|+-
  Sum6 : Sum  Inputs=+++
  Tm*' : Outport  VectorParamsAs1DForOutWhenUnconnected=off
  wires:
  Gain8/1 -> Sum6/2
  Gain9/1 -> Sum6/1
  omega_m/1 -> Sum5/2
  Gain7/1 -> Sum6/3
  Sum6/1 -> Tm*'/1  "Tm*'"
  Discrete-Time Integrator/1 -> Discrete-Time Integrator1/1, Gain8/1
  Discrete-Time Integrator1/1 -> Gain9/1
  Sum5/1 -> Discrete-Time Integrator/1, Gain7/1  "e_w"
  omega_m*/1 -> Sum5/1

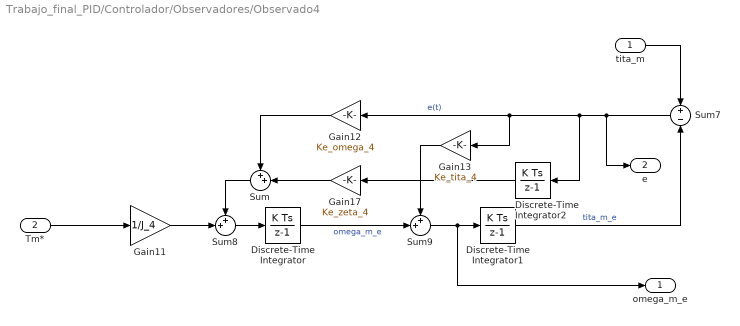
== system Trabajo_final_PID/Controlador/Observadores/Observado4 ==
  tita_m : Inport
  Tm* : Inport  Port=2
  Discrete-Time Integrator : DiscreteIntegrator  SampleTime=Ts2  ICPrevOutput=DiscIntNeverNeededParam  ICPrevScaledInput=DiscIntNeverNeededParam
  Discrete-Time Integrator1 : DiscreteIntegrator  SampleTime=Ts2  ICPrevOutput=DiscIntNeverNeededParam  ICPrevScaledInput=DiscIntNeverNeededParam
  Discrete-Time Integrator2 : DiscreteIntegrator  SampleTime=Ts2  ICPrevOutput=DiscIntNeverNeededParam  ICPrevScaledInput=DiscIntNeverNeededParam
  Gain11 : Gain  Gain=1/J_4
  Gain12 : Gain  Gain=Ke_omega_4
  Gain13 : Gain  Gain=Ke_tita_4
  Gain17 : Gain  Gain=Ke_zeta_4
  Sum : Sum  Inputs=++|
  Sum7 : Sum  Inputs=+-
  Sum8 : Sum  Inputs=++|
  Sum9 : Sum  Inputs=++|
  omega_m_e : Outport  VectorParamsAs1DForOutWhenUnconnected=off
  e : Outport  Port=2
  wires:
  Gain11/1 -> Sum8/2
  Discrete-Time Integrator/1 -> Sum9/2  "omega_m_e"
  Discrete-Time Integrator1/1 -> Sum7/2  "tita_m_e"
  tita_m/1 -> Sum7/1
  Discrete-Time Integrator2/1 -> Gain17/1
  Sum8/1 -> Discrete-Time Integrator/1
  Gain13/1 -> Sum9/1
  Sum7/1 -> e/1, Discrete-Time Integrator2/1, Gain13/1, Gain12/1  "e(t)"
  Sum9/1 -> omega_m_e/1, Discrete-Time Integrator1/1
  Gain17/1 -> Sum/2
  Gain12/1 -> Sum/1
  Sum/1 -> Sum8/1
  Tm*/1 -> Gain11/1

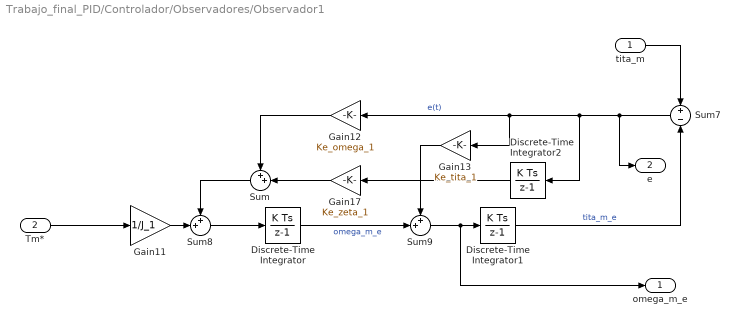
== system Trabajo_final_PID/Controlador/Observadores/Observador1 ==
  tita_m : Inport
  Tm* : Inport  Port=2
  Discrete-Time Integrator : DiscreteIntegrator  SampleTime=Ts2  ICPrevOutput=DiscIntNeverNeededParam  ICPrevScaledInput=DiscIntNeverNeededParam
  Discrete-Time Integrator1 : DiscreteIntegrator  SampleTime=Ts2  ICPrevOutput=DiscIntNeverNeededParam  ICPrevScaledInput=DiscIntNeverNeededParam
  Discrete-Time Integrator2 : DiscreteIntegrator  SampleTime=Ts2  ICPrevOutput=DiscIntNeverNeededParam  ICPrevScaledInput=DiscIntNeverNeededParam
  Gain11 : Gain  Gain=1/J_1
  Gain12 : Gain  Gain=Ke_omega_1
  Gain13 : Gain  Gain=Ke_tita_1
  Gain17 : Gain  Gain=Ke_zeta_1
  Sum : Sum  Inputs=++|
  Sum7 : Sum  Inputs=+-
  Sum8 : Sum  Inputs=++|
  Sum9 : Sum  Inputs=++|
  omega_m_e : Outport  VectorParamsAs1DForOutWhenUnconnected=off
  e : Outport  Port=2
  wires:
  Gain11/1 -> Sum8/2
  Discrete-Time Integrator/1 -> Sum9/2  "omega_m_e"
  Discrete-Time Integrator1/1 -> Sum7/2  "tita_m_e"
  tita_m/1 -> Sum7/1
  Discrete-Time Integrator2/1 -> Gain17/1
  Sum8/1 -> Discrete-Time Integrator/1
  Gain13/1 -> Sum9/1
  Sum7/1 -> e/1, Discrete-Time Integrator2/1, Gain13/1, Gain12/1  "e(t)"
  Sum9/1 -> omega_m_e/1, Discrete-Time Integrator1/1
  Gain17/1 -> Sum/2
  Gain12/1 -> Sum/1
  Sum/1 -> Sum8/1
  Tm*/1 -> Gain11/1

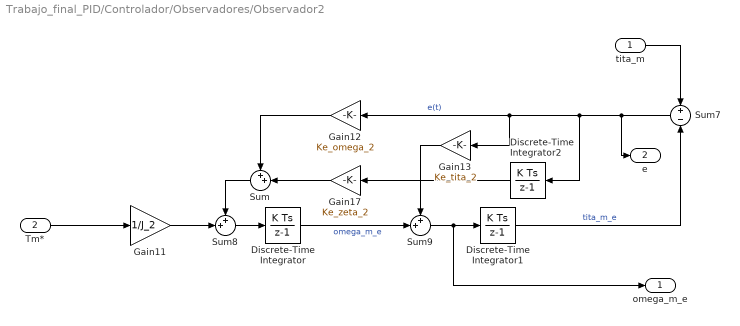
== system Trabajo_final_PID/Controlador/Observadores/Observador2 ==
  tita_m : Inport
  Tm* : Inport  Port=2
  Discrete-Time Integrator : DiscreteIntegrator  SampleTime=Ts2  ICPrevOutput=DiscIntNeverNeededParam  ICPrevScaledInput=DiscIntNeverNeededParam
  Discrete-Time Integrator1 : DiscreteIntegrator  SampleTime=Ts2  ICPrevOutput=DiscIntNeverNeededParam  ICPrevScaledInput=DiscIntNeverNeededParam
  Discrete-Time Integrator2 : DiscreteIntegrator  SampleTime=Ts2  ICPrevOutput=DiscIntNeverNeededParam  ICPrevScaledInput=DiscIntNeverNeededParam
  Gain11 : Gain  Gain=1/J_2
  Gain12 : Gain  Gain=Ke_omega_2
  Gain13 : Gain  Gain=Ke_tita_2
  Gain17 : Gain  Gain=Ke_zeta_2
  Sum : Sum  Inputs=++|
  Sum7 : Sum  Inputs=+-
  Sum8 : Sum  Inputs=++|
  Sum9 : Sum  Inputs=++|
  omega_m_e : Outport  VectorParamsAs1DForOutWhenUnconnected=off
  e : Outport  Port=2
  wires:
  Gain11/1 -> Sum8/2
  Discrete-Time Integrator/1 -> Sum9/2  "omega_m_e"
  Discrete-Time Integrator1/1 -> Sum7/2  "tita_m_e"
  tita_m/1 -> Sum7/1
  Discrete-Time Integrator2/1 -> Gain17/1
  Sum8/1 -> Discrete-Time Integrator/1
  Gain13/1 -> Sum9/1
  Sum7/1 -> e/1, Discrete-Time Integrator2/1, Gain13/1, Gain12/1  "e(t)"
  Sum9/1 -> omega_m_e/1, Discrete-Time Integrator1/1
  Gain17/1 -> Sum/2
  Gain12/1 -> Sum/1
  Sum/1 -> Sum8/1
  Tm*/1 -> Gain11/1

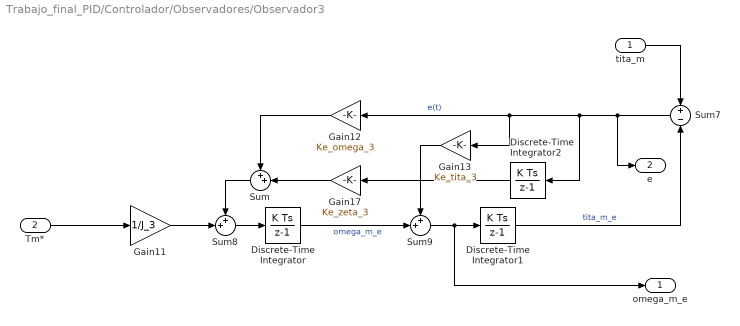
== system Trabajo_final_PID/Controlador/Observadores/Observador3 ==
  tita_m : Inport
  Tm* : Inport  Port=2
  Discrete-Time Integrator : DiscreteIntegrator  SampleTime=Ts2  ICPrevOutput=DiscIntNeverNeededParam  ICPrevScaledInput=DiscIntNeverNeededParam
  Discrete-Time Integrator1 : DiscreteIntegrator  SampleTime=Ts2  ICPrevOutput=DiscIntNeverNeededParam  ICPrevScaledInput=DiscIntNeverNeededParam
  Discrete-Time Integrator2 : DiscreteIntegrator  SampleTime=Ts2  ICPrevOutput=DiscIntNeverNeededParam  ICPrevScaledInput=DiscIntNeverNeededParam
  Gain11 : Gain  Gain=1/J_3
  Gain12 : Gain  Gain=Ke_omega_3
  Gain13 : Gain  Gain=Ke_tita_3
  Gain17 : Gain  Gain=Ke_zeta_3
  Sum : Sum  Inputs=++|
  Sum7 : Sum  Inputs=+-
  Sum8 : Sum  Inputs=++|
  Sum9 : Sum  Inputs=++|
  omega_m_e : Outport  VectorParamsAs1DForOutWhenUnconnected=off
  e : Outport  Port=2
  wires:
  Gain11/1 -> Sum8/2
  Discrete-Time Integrator/1 -> Sum9/2  "omega_m_e"
  Discrete-Time Integrator1/1 -> Sum7/2  "tita_m_e"
  tita_m/1 -> Sum7/1
  Discrete-Time Integrator2/1 -> Gain17/1
  Sum8/1 -> Discrete-Time Integrator/1
  Gain13/1 -> Sum9/1
  Sum7/1 -> e/1, Discrete-Time Integrator2/1, Gain13/1, Gain12/1  "e(t)"
  Sum9/1 -> omega_m_e/1, Discrete-Time Integrator1/1
  Gain17/1 -> Sum/2
  Gain12/1 -> Sum/1
  Sum/1 -> Sum8/1
  Tm*/1 -> Gain11/1
